simulink model "s7segm_top"  (R2017b)
settings: Solver=VariableStepAuto  StartTime=0.0  StopTime=2  RelTol=1e-3
libraries: simulink x1
settings Model: Creator=criedl  LastModifiedBy=criedl
settings DataIOCC: ReturnWorkspaceOutputs=on
settings DebuggingCC: SFMachineParentedDataDiag=error
settings SFSimCC: SimUseLocalCustomCode=on
settings RTWCC: RTWUseLocalCustomCode=on

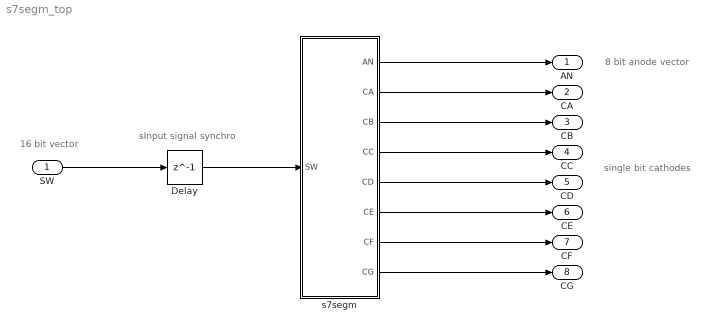
== system s7segm_top ==
  note: 8 bit anode vector
  note: single bit cathodes
  note: sInput signal synchro
  note: 16 bit vector
  SW : Inport  OutDataTypeStr=fixdt(0,16,0)
  Delay : Delay  DelayLength=1  InitialCondition=0
  s7segm : Subsystem
  AN : Outport  InitialOutput=0  VectorParamsAs1DForOutWhenUnconnected=on
  CA : Outport  Port=2  InitialOutput=0  VectorParamsAs1DForOutWhenUnconnected=on
  CB : Outport  Port=3  InitialOutput=0  VectorParamsAs1DForOutWhenUnconnected=on
  CC : Outport  Port=4  InitialOutput=0  VectorParamsAs1DForOutWhenUnconnected=on
  CD : Outport  Port=5  InitialOutput=0  VectorParamsAs1DForOutWhenUnconnected=on
  CE : Outport  Port=6  InitialOutput=0  VectorParamsAs1DForOutWhenUnconnected=on
  CF : Outport  Port=7  InitialOutput=0  VectorParamsAs1DForOutWhenUnconnected=on
  CG : Outport  Port=8  InitialOutput=0  VectorParamsAs1DForOutWhenUnconnected=on
  wires:
  s7segm/1(AN) -> AN/1
  s7segm/7(CF) -> CF/1
  s7segm/6(CE) -> CE/1
  s7segm/8(CG) -> CG/1
  s7segm/2(CA) -> CA/1
  s7segm/4(CC) -> CC/1
  s7segm/5(CD) -> CD/1
  s7segm/3(CB) -> CB/1
  SW/1 -> Delay/1
  Delay/1 -> s7segm/1(SW)

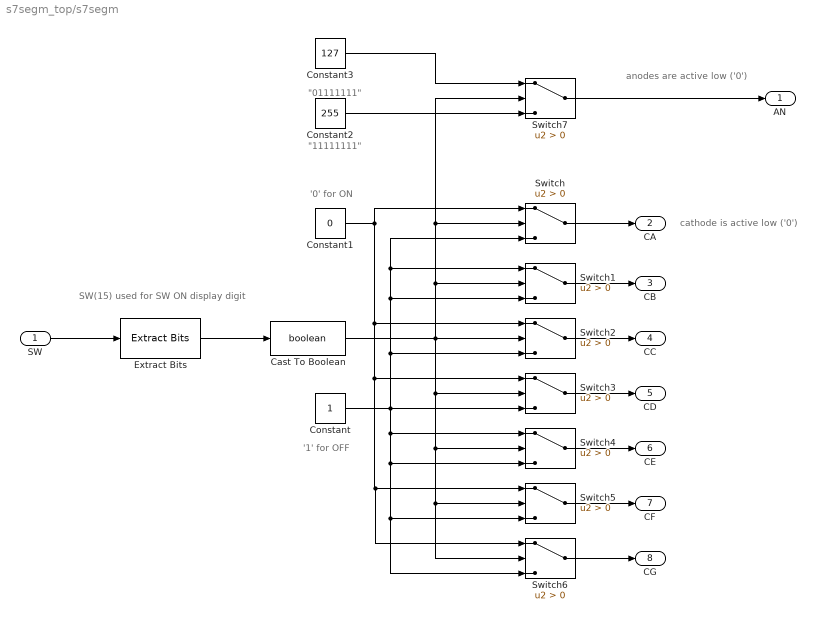
== system s7segm_top/s7segm ==
  note: '0' for ON
  note: SW(15) used for SW ON display digit
  note: '1' for OFF
  note: "11111111"
  note: "01111111"
  note: anodes are active low ('0')
  note: cathode is active low ('0')
  SW : Inport
  Cast To Boolean : DataTypeConversion  OutDataTypeStr=boolean
  Constant : Constant  OutDataTypeStr=boolean
  Constant1 : Constant  Value=0  OutDataTypeStr=boolean
  Constant2 : Constant  Value=255  OutDataTypeStr=fixdt(0,8,0)
  Constant3 : Constant  Value=127  OutDataTypeStr=fixdt(0,8,0)
  Extract Bits : simulink/Logic and Bit Operations/Extract Bits  bitsToExtract=Range of bits  numBits=8  bitIdxRange=[15 15]  outScalingMode=Preserve fixed-point scaling
  Switch{,1..7} (8 alike) : Switch  Criteria=u2 > Threshold
  AN : Outport  OutDataTypeStr=fixdt(0,8,0)  VectorParamsAs1DForOutWhenUnconnected=on
  CA : Outport  Port=2  VectorParamsAs1DForOutWhenUnconnected=on
  CB : Outport  Port=3  VectorParamsAs1DForOutWhenUnconnected=on
  CC : Outport  Port=4  VectorParamsAs1DForOutWhenUnconnected=on
  CD : Outport  Port=5  VectorParamsAs1DForOutWhenUnconnected=on
  CE : Outport  Port=6  VectorParamsAs1DForOutWhenUnconnected=on
  CF : Outport  Port=7  VectorParamsAs1DForOutWhenUnconnected=on
  CG : Outport  Port=8  VectorParamsAs1DForOutWhenUnconnected=on
  wires:
  Constant2/1 -> Switch7/3
  Constant1/1 -> Switch2/1, Switch3/1, Switch6/1, Switch5/1, Switch/1
  Constant/1 -> Switch1/1, Switch/3, Switch1/3, Switch2/3, Switch3/3, Switch4/1, Switch4/3, Switch5/3, Switch6/3
  Cast To Boolean/1 -> Switch6/2, Switch5/2, Switch4/2, Switch3/2, Switch2/2, Switch1/2, Switch7/2, Switch/2
  Switch3/1 -> CD/1
  Switch6/1 -> CG/1
  Constant3/1 -> Switch7/1
  Extract Bits/1 -> Cast To Boolean/1
  Switch/1 -> CA/1
  Switch4/1 -> CE/1
  Switch2/1 -> CC/1
  Switch1/1 -> CB/1
  Switch5/1 -> CF/1
  Switch7/1 -> AN/1
  SW/1 -> Extract Bits/1
